simulink library "sm_boom_lift_crawler_lib_actuators"  (R2026a)
settings: Solver=ode23t
undefined symbols (not defined in the file): actuators, BasketR, cylinders, Extend, Jib, LevelM, LevelS, Lift, lines, OutFL, OutFR, OutRL, OutRR, Tilt, TrackL, TrackR, Turret, valves
libraries: SimscapeFluids_lib x92, fl_lib x67, sm_boom_lift_crawler_lib x24, nesl_utility x13, Custom_Valves x2
(part 5 of 5)

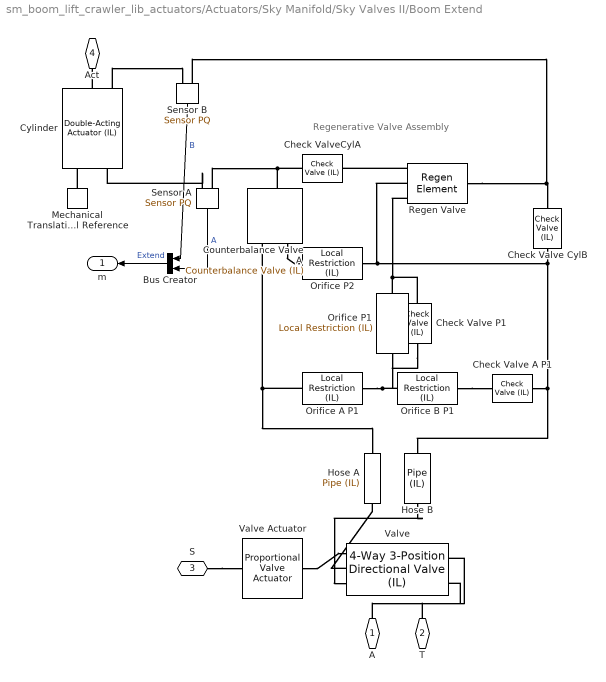
== system sm_boom_lift_crawler_lib_actuators/Actuators/Sky Manifold/Sky Valves II/Boom Extend ==
  note: Regenerative Valve Assembly
  Bus Creator : BusCreator  Inputs=2
  Check Valve P1 : SimscapeFluids_lib/Isothermal Liquid/Valves & Orifices/Directional Control Valves/Check Valve (IL)  opening_spec=fluids.isothermal_liquid.valves_orifices.enum.PressureOpeningSpec.Linear  pressure_control_spec=fluids.isothermal_liquid.valves_orifices.enum.pressure_control_spec.dp  p_crack_differential=valves.check.p.crack psi  p_crack_gauge=0.1 MPa  press_max_differential=valves.check.p.max psi  press_max_gauge=0.2 MPa  area_max=orifices.sky.rg.s in^2  area_leak=1e-12 m^2  p_diff_TLU=[0.01 : 0.01 : 0.1] MPa  valve_area_TLU=[1e-10, 1e-05, 2e-05, 3e-05, 4e-05, 5e-05, 6e-05, 7.5e-05, 8.5e-05, .0001] m^2  vol_flow_TLU=[.000358, .045, .11, .191, .284, .39, .505, .63, .764, .905] .* 1e-3 m^3/s  area=inf m^2  Cd=0.7  Re_c=150  smoothing_factor=0  pressure_recovery=false  opening_dynamics=1  tau=0.1 s
  Check Valve A P1 : SimscapeFluids_lib/Isothermal Liquid/Valves & Orifices/Directional Control Valves/Check Valve (IL)  opening_spec=fluids.isothermal_liquid.valves_orifices.enum.PressureOpeningSpec.Linear  pressure_control_spec=fluids.isothermal_liquid.valves_orifices.enum.pressure_control_spec.dp  p_crack_differential=valves.check.p.crack psi  p_crack_gauge=0.1 MPa  press_max_differential=valves.check.p.max psi  press_max_gauge=0.2 MPa  area_max=orifices.sky.r2.s in^2  area_leak=1e-12 m^2  p_diff_TLU=[0.01 : 0.01 : 0.1] MPa  valve_area_TLU=[1e-10, 1e-05, 2e-05, 3e-05, 4e-05, 5e-05, 6e-05, 7.5e-05, 8.5e-05, .0001] m^2  vol_flow_TLU=[.000358, .045, .11, .191, .284, .39, .505, .63, .764, .905] .* 1e-3 m^3/s  area=inf m^2  Cd=0.7  Re_c=150  smoothing_factor=0  pressure_recovery=false  opening_dynamics=1  tau=0.1 s
  Check Valve CylB : SimscapeFluids_lib/Isothermal Liquid/Valves & Orifices/Directional Control Valves/Check Valve (IL)  opening_spec=fluids.isothermal_liquid.valves_orifices.enum.PressureOpeningSpec.Linear  pressure_control_spec=fluids.isothermal_liquid.valves_orifices.enum.pressure_control_spec.dp  p_crack_differential=valves.check.p.crack psi  p_crack_gauge=0.1 MPa  press_max_differential=valves.check.p.max psi  press_max_gauge=0.2 MPa  area_max=lines.sky.c3.d.b in^2  area_leak=1e-12 m^2  p_diff_TLU=[0.01 : 0.01 : 0.1] MPa  valve_area_TLU=[1e-10, 1e-05, 2e-05, 3e-05, 4e-05, 5e-05, 6e-05, 7.5e-05, 8.5e-05, .0001] m^2  vol_flow_TLU=[.000358, .045, .11, .191, .284, .39, .505, .63, .764, .905] .* 1e-3 m^3/s  area=inf m^2  Cd=0.7  Re_c=150  smoothing_factor=0  pressure_recovery=false  opening_dynamics=0  tau=0.1 s
  Check ValveCylA : SimscapeFluids_lib/Isothermal Liquid/Valves & Orifices/Directional Control Valves/Check Valve (IL)  opening_spec=fluids.isothermal_liquid.valves_orifices.enum.PressureOpeningSpec.Linear  pressure_control_spec=fluids.isothermal_liquid.valves_orifices.enum.pressure_control_spec.dp  p_crack_differential=valves.check.p.crack psi  p_crack_gauge=0.1 MPa  press_max_differential=valves.check.p.max psi  press_max_gauge=0.2 MPa  area_max=lines.sky.c3.s.a in^2  area_leak=1e-12 m^2  p_diff_TLU=[0.01 : 0.01 : 0.1] MPa  valve_area_TLU=[1e-10, 1e-05, 2e-05, 3e-05, 4e-05, 5e-05, 6e-05, 7.5e-05, 8.5e-05, .0001] m^2  vol_flow_TLU=[.000358, .045, .11, .191, .284, .39, .505, .63, .764, .905] .* 1e-3 m^3/s  area=inf m^2  Cd=0.7  Re_c=150  smoothing_factor=0  pressure_recovery=false  opening_dynamics=1  tau=0.1 s
  Counterbalance Valve A : SimscapeFluids_lib/Isothermal Liquid/Valves & Orifices/Pressure Control Valves/Counterbalance Valve (IL)  opening_spec=1  p_set_diff=valves.counterbalance.c3.ps psi  p_max_diff=(valves.counterbalance.c3.k)*(valves.control.l.max) + (valves.counterbalance.c3.ps) psi  area_max=lines.sky.c3.s.a in^2  area_leak=1e-9 in^2  p_diff_TLU=39.3701*(valves.counterbalance.c3.k)*([-.002, 0, .005, .015]) + (valves.counterbalance.c3.ps) psi  valve_area_TLU=[1e-09, 4e-09, 1e-05, 1.02e-05] m^2  p_diff_TLU_ref=5 : 0.2 : 6 MPa  vol_flow_TLU_ref=[6.4e-09, .0013, .0027, .0041, .0055, .007] m^3/s  pilot_ratio=valves.counterbalance.c3.pr  back_ratio=valves.counterbalance.c3.pbr  Cd=0.7  Re_c=150  smoothing_factor=0  opening_dynamics=1  tau=valves.counterbalance.common.tau s  check_p_crack=valves.counterbalance.common.pc psi  check_p_max=valves.counterbalance.common.pm psi  check_area_max=lines.sky.c3.s.a in^2  check_p_diff_TLU=[0.01 : 0.01 : 0.1] MPa  check_area_TLU=[1e-10, 1e-05, 2e-05, 3e-05, 4e-05, 5e-05, 6e-05, 7.5e-05, 8.5e-05, .0001] m^2  check_vol_flow_TLU=[.000358, .045, .11, .191, .284, .39, .505, .63, .764, .905] .* 1e-3 m^3/s
  Cylinder : SimscapeFluids_lib/Isothermal Liquid/Actuators/Double-Acting Actuator (IL)  single_fluid=true  mech_orientation=1  piston_area_A=cylinders.sky.c3.s.a in^2  piston_area_B=cylinders.sky.c3.s.b in^2  stroke=cylinders.sky.c3.stroke in  dead_volume_A=cylinders.sky.c3.v.dead in^3  dead_volume_B=cylinders.sky.c3.v.dead in^3  pressure_spec=foundation.enum.pressure_spec.atmospheric  environment_pressure=0.101325 MPa  hardstop_model=1  stiff_coeff=cylinders.sky.c3.stops.kc N/m  damping_coeff=cylinders.sky.c3.stops.bc N/(m/s)  transition=1 mm  coeff_rest=0.7  v_tol=0.001 m/s  f_tol=0.001 N  cushion_A_spec=false  area_plunger_A=1e-4 m^2  length_plunger_A=1e-3 m  area_cushion_orifice_A=1e-6 m^2  area_leak_plunger_A=1e-7 m^2  p_crack_differential_A=0.01 MPa  press_max_differential_A=0.1 MPa  check_valve_area_max_A=1e-4 m^2  check_valve_area_leak_A=1e-10 m^2  smoothing_factor_A=0  cushion_B_spec=false  area_plunger_B=1e-4 m^2  length_plunger_B=1e-3 m  area_cushion_orifice_B=1e-6 m^2  area_leak_plunger_B=1e-7 m^2  p_crack_differential_B=0.01 MPa  press_max_differential_B=0.1 MPa  check_valve_area_max_B=1e-4 m^2  check_valve_area_leak_B=1e-10 m^2  smoothing_factor_B=0  friction_spec=false  breakaway_Coulomb_ratio=1.2  breakaway_velocity=0.1 m/s  preload_force=20 N  Coulomb_coeff=1e-6 N/Pa  viscous_coeff=100 N*s/m  leakage_spec=false  clearance=1e-4 m  piston_length=0.01 m  displacement_spec=foundation.enum.DisplacementSpec.Calculate  x0=0 in  dynamic_compressibility=true  p0_A=lines.sky.c3.p0.a + 14.6959 psi  p0_B=lines.sky.c3.p0.b + 14.6959 psi  p_nominal_A=0.101325 MPa  p_nominal_B=0.101325 MPa
      settings: LogSimulationData=on
  Hose A : SimscapeFluids_lib/Isothermal Liquid/Pipes & Fittings/Pipe (IL)  dynamic_compressibility=true  inertia=false  num_segments=1  pipe_length=lines.sky.c3.l ft  cross_section_geometry=fluids.isothermal_liquid.pipes_fittings.enum.cross_section_geometry.circular  pipe_diameter=lines.sky.c3.d.a in  pipe_inner_diameter=0.05 m  pipe_outer_diameter=0.1 m  pipe_width=0.1 m  pipe_height=0.1 m  pipe_major_axis=0.1 m  pipe_minor_axis=0.05 m  pipe_side=0.1 m  pipe_angle=30 deg  pipe_area=1e-4 m^2  Dh=1.12e-2 m  elevation_spec=foundation.enum.constant_variable.constant  elevation_gain=0 m  gravity_spec=foundation.enum.constant_variable.constant  g=9.81 m/s^2  pressure_loss_spec=fluids.isothermal_liquid.pipes_fittings.enum.pressure_loss_spec.haaland  mdot_nominal=[.1, 1] kg/s  p_diff_nominal=[.001, .01] MPa  mdot_threshold=1e-6 kg/s  local_pressure_loss_spec=fluids.isothermal_liquid.pipes_fittings.enum.local_loss_spec.aggregate_length  length_add=lines.sky.c3.lr ft  loss_coefficient=0.1  roughness_spec=fluids.isothermal_liquid.pipes_fittings.enum.roughness_spec.custom  roughness=15e-6 m  Re_friction_TLU=[400, 1000, 1500, 3000, 4000, 6000, 10000, 20000, 40000, 60000, 100000, 100000000]  friction_factor_TLU=[.264, .112, .071, .0417, .0387, .0268, .025, .0232, .0226, .022, .0214, .0214]  Re_lam=2000  Re_tur=4000  shape_factor=64  pipe_wall_spec=fluids.isothermal_liquid.pipes_fittings.enum.wall_spec.rigid  vol_expansion_spec=fluids.isothermal_liquid.pipes_fittings.enum.vol_expansion_spec.area  area_pressure_gain=1e-6 m^2/MPa  static_pressure_TLU=[.1, 1] MPa  area_pressure_gain_TLU=[1e-05, 1.1e-05] m^2  material_behavior_spec=fluids.isothermal_liquid.pipes_fittings.enum.PipeMaterialBehavior.Linear  diameter_pressure_gain=2e-12 m/Pa  wall_thickness=0.05 m  elastic_modulus=69 GPa  stress_TLU=[276, 310] MPa  strain_TLU=[.004, .02]  stress_assert_action=simscape.enum.assert.action.none  stress_max=400 MPa  poisson_ratio=0.33  wall_time_constant=0.01 s  p0=lines.sky.c3.p0.a + 14.6959 psi  mdot0=0 kg/s
  Hose B : SimscapeFluids_lib/Isothermal Liquid/Pipes & Fittings/Pipe (IL)  dynamic_compressibility=true  inertia=false  num_segments=1  pipe_length=lines.sky.c3.l ft  cross_section_geometry=fluids.isothermal_liquid.pipes_fittings.enum.cross_section_geometry.circular  pipe_diameter=lines.sky.c3.d.b in  pipe_inner_diameter=0.05 m  pipe_outer_diameter=0.1 m  pipe_width=0.1 m  pipe_height=0.1 m  pipe_major_axis=0.1 m  pipe_minor_axis=0.05 m  pipe_side=0.1 m  pipe_angle=30 deg  pipe_area=1e-4 m^2  Dh=1.12e-2 m  elevation_spec=foundation.enum.constant_variable.constant  elevation_gain=0 m  gravity_spec=foundation.enum.constant_variable.constant  g=9.81 m/s^2  pressure_loss_spec=fluids.isothermal_liquid.pipes_fittings.enum.pressure_loss_spec.haaland  mdot_nominal=[.1, 1] kg/s  p_diff_nominal=[.001, .01] MPa  mdot_threshold=1e-6 kg/s  local_pressure_loss_spec=fluids.isothermal_liquid.pipes_fittings.enum.local_loss_spec.aggregate_length  length_add=lines.sky.c3.lr ft  loss_coefficient=0.1  roughness_spec=fluids.isothermal_liquid.pipes_fittings.enum.roughness_spec.custom  roughness=15e-6 m  Re_friction_TLU=[400, 1000, 1500, 3000, 4000, 6000, 10000, 20000, 40000, 60000, 100000, 100000000]  friction_factor_TLU=[.264, .112, .071, .0417, .0387, .0268, .025, .0232, .0226, .022, .0214, .0214]  Re_lam=2000  Re_tur=4000  shape_factor=64  pipe_wall_spec=fluids.isothermal_liquid.pipes_fittings.enum.wall_spec.rigid  vol_expansion_spec=fluids.isothermal_liquid.pipes_fittings.enum.vol_expansion_spec.area  area_pressure_gain=1e-6 m^2/MPa  static_pressure_TLU=[.1, 1] MPa  area_pressure_gain_TLU=[1e-05, 1.1e-05] m^2  material_behavior_spec=fluids.isothermal_liquid.pipes_fittings.enum.PipeMaterialBehavior.Linear  diameter_pressure_gain=2e-12 m/Pa  wall_thickness=0.05 m  elastic_modulus=69 GPa  stress_TLU=[276, 310] MPa  strain_TLU=[.004, .02]  stress_assert_action=simscape.enum.assert.action.none  stress_max=400 MPa  poisson_ratio=0.33  wall_time_constant=0.01 s  p0=lines.sky.c3.p0.b + 14.6959 psi  mdot0=0 kg/s
  Mechanical Translational Reference : fl_lib/Mechanical/Translational Elements/Mechanical Translational Reference
  Orifice A P1 : fl_lib/Isothermal Liquid/Elements/Local Restriction (IL)  restriction_type=1  restriction_area=orifices.sky.rg.s in^2  min_area=1e-10 m^2  max_area=0.005 m^2  area=inf in^2  Cd=0.7  Re_c=150  pressure_recovery=simscape.enum.onoff.off
  Orifice B P1 : fl_lib/Isothermal Liquid/Elements/Local Restriction (IL)  restriction_type=1  restriction_area=orifices.sky.rg.s in^2  min_area=1e-10 m^2  max_area=0.005 m^2  area=inf in^2  Cd=0.7  Re_c=150  pressure_recovery=simscape.enum.onoff.off
  Orifice P1 : fl_lib/Isothermal Liquid/Elements/Local Restriction (IL)  restriction_type=1  restriction_area=orifices.sky.rg.s in^2  min_area=1e-10 m^2  max_area=0.005 m^2  area=inf in^2  Cd=0.7  Re_c=150  pressure_recovery=simscape.enum.onoff.off
  Orifice P2 : fl_lib/Isothermal Liquid/Elements/Local Restriction (IL)  restriction_type=1  restriction_area=orifices.sky.rg.s in^2  min_area=1e-10 m^2  max_area=0.005 m^2  area=inf in^2  Cd=0.7  Re_c=150  pressure_recovery=simscape.enum.onoff.off
  Regen Valve : Custom_Valves/Regen Element  sMax=valves.control.l.max  T=0.1  pCrack=1450  pMax=1550  AMax=lines.sky.c3.s.a  kA=1  kP1=3  kP2=1
  Sensor A : sm_boom_lift_crawler_lib/Sensor PQ  SystemSampleTime=-1  VariantActivationTime=update diagram  EmptyChoice=off  PassThrough=off  PassThroughVariantControl=(default)  EmptyChoiceVariantControl=(default)  AllowFlexibleInterface=on  Latency=0  AutoFrameSizeCalculation=off
  Sensor B : sm_boom_lift_crawler_lib/Sensor PQ  SystemSampleTime=-1  VariantActivationTime=update diagram  EmptyChoice=off  PassThrough=off  PassThroughVariantControl=(default)  EmptyChoiceVariantControl=(default)  AllowFlexibleInterface=on  Latency=0  AutoFrameSizeCalculation=off
  Valve : SimscapeFluids_lib/Isothermal Liquid/Valves & Orifices/Directional Control Valves/4-Way 3-Position Directional Valve (IL)  open_orifices_pos=fluids.isothermal_liquid.valves_orifices.directional_control_valves.enum.directional_valve_open_orifices_pos_neg.PA_BT  open_orifices_neu=fluids.isothermal_liquid.valves_orifices.directional_control_valves.enum.directional_valve_open_orifices_neutral.all_closed  open_orifices_neg=fluids.isothermal_liquid.valves_orifices.directional_control_valves.enum.directional_valve_open_orifices_pos_neg.PB_AT  neutral_assert_action=0  area_spec=fluids.isothermal_liquid.valves_orifices.directional_control_valves.enum.directional_valve_area_spec.different  valve_spec=1  del_S_max=(valves.control.l.max) - (valves.control.l.max)/(lines.sky.r1.s)*(1e-9) in  area_max=lines.sky.r1.s in^2  del_S_TLU=[0, .00125, .0025, .00375, .005] m  valve_area_TLU=[1e-09, 2.0352e-07, 4.0736e-05, .00011438, .00034356] m^2  del_S_vol_flow_TLU=[0, .00125, .0025, .00375, .005] m  p_diff_TLU=[-10000000, -5000000, -2000000, 2000000, 5000000, 10000000] Pa  vol_flow_TLU=[-1e-07, -7.0711e-08, -4.4721e-08, 4.4721e-08, 7.0711e-08, 1e-07; -2.0352e-05, -1.4391e-05, -9.1017e-06, 9.1017e-06, 1.4391e-05, 2.0352e-05; -.0040736, -.0028805, -.0018218, .0018218, .0028805, .0040736; -.011438, -.0080879, -.0051152, .0051152, .0080879, .011438; -.034356, -.024293, -.015364, .015364, .024293, .034356] m^3/s  p_diff_TLU_const=[-.1, .3, .5, .7] MPa  vol_flow_TLU_const=[-.0009, .0016, .002, .0024] m^3/s  area_const=1e-4 m^2  area_leak=1e-9 in^2  area=inf m^2  Cd=0.7  Re_c=150  smoothing_factor=0.01  pressure_recovery=false  S_max_PA=-(0) + 0.0254*(valves.control.l.max) m  del_S_max_PA=(valves.control.l.max) - (valves.control.l.max)/(lines.sky.c3.s.a)*(1e-9) in  area_max_PA=lines.sky.c3.s.a in^2  del_S_TLU_PA=[0, .00125, .0025, .00375, .005] m  valve_area_TLU_PA=[1e-09, 2.0352e-07, 4.0736e-05, .00011438, .00034356] m^2  del_S_vol_flow_TLU_PA=[0, .00125, .0025, .00375, .005] m  p_diff_TLU_PA=[-10000000, -5000000, -2000000, 2000000, 5000000, 10000000] Pa  vol_flow_TLU_PA=[-1e-07, -7.0711e-08, -4.4721e-08, 4.4721e-08, 7.0711e-08, 1e-07; -2.0352e-05, -1.4391e-05, -9.1017e-06, 9.1017e-06, 1.4391e-05, 2.0352e-05; -.0040736, -.0028805, -.0018218, .0018218, .0028805, .0040736; -.011438, -.0080879, -.0051152, .0051152, .0080879, .011438; -.034356, -.024293, -.015364, .015364, .024293, .034356] m^3/s  area_const_PA=1e-4 m^2  p_diff_TLU_const_PA=[-.1, .3, .5, .7] MPa  vol_flow_TLU_const_PA=[-.0009, .0016, .002, .0024] m^3/s  S_max_PB=(0) - 0.0254*(valves.control.l.max) m  del_S_max_PB=(valves.control.l.max) - (valves.control.l.max)/(lines.sky.c3.s.b)*(1e-9) in  area_max_PB=lines.sky.c3.s.b in^2  del_S_TLU_PB=[0, .00125, .0025, .00375, .005] m  valve_area_TLU_PB=[1e-09, 2.0352e-07, 4.0736e-05, .00011438, .00034356] m^2  del_S_vol_flow_TLU_PB=[0, .00125, .0025, .00375, .005] m  p_diff_TLU_PB=[-10000000, -5000000, -2000000, 2000000, 5000000, 10000000] Pa  vol_flow_TLU_PB=[-1e-07, -7.0711e-08, -4.4721e-08, 4.4721e-08, 7.0711e-08, 1e-07; -2.0352e-05, -1.4391e-05, -9.1017e-06, 9.1017e-06, 1.4391e-05, 2.0352e-05; -.0040736, -.0028805, -.0018218, .0018218, .0028805, .0040736; -.011438, -.0080879, -.0051152, .0051152, .0080879, .011438; -.034356, -.024293, -.015364, .015364, .024293, .034356] m^3/s  area_const_PB=1e-4 m^2  p_diff_TLU_const_PB=[-.1, .3, .5, .7] MPa  vol_flow_TLU_const_PB=[-.0009, .0016, .002, .0024] m^3/s  S_max_AB=7.5e-3 m  del_S_max_AB=0.005 m  area_max_AB=1e-4 m^2  del_S_TLU_AB=[0, .00125, .0025, .00375, .005] m  valve_area_TLU_AB=[1e-10, 1e-05, 4e-05, 6e-05, .0001] m^2  del_S_vol_flow_TLU_AB=[0, .00125, .0025, .00375, .005] m  p_diff_TLU_AB=[-.1, .3, .5, .7] MPa  vol_flow_TLU_AB=[-1e-08, 2.2e-08, 2.8e-08, 3.4e-08; -9e-06, .00015, .0002, .00024; -.00036, .00063, .00081, .00096; -.00054, .00094, .0012, .0014; -.00091, .0016, .002, .0024] m^3/s  area_const_AB=1e-4 m^2  p_diff_TLU_const_AB=[-.1, .3, .5, .7] MPa  vol_flow_TLU_const_AB=[-.0009, .0016, .002, .0024] m^3/s  S_max_AT=(0) - 0.0254*(valves.control.l.max) m  del_S_max_AT=(valves.control.l.max) - (valves.control.l.max)/(lines.sky.main.s.t)*(1e-9) in  area_max_AT=lines.sky.main.s.t in^2  del_S_TLU_AT=[0, .00125, .0025, .00375, .005] m  valve_area_TLU_AT=[1e-09, 2.0352e-07, 4.0736e-05, .00011438, .00034356] m^2  del_S_vol_flow_TLU_AT=[0, .00125, .0025, .00375, .005] m  p_diff_TLU_AT=[-10000000, -5000000, -2000000, 2000000, 5000000, 10000000] Pa  vol_flow_TLU_AT=[-1e-07, -7.0711e-08, -4.4721e-08, 4.4721e-08, 7.0711e-08, 1e-07; -2.0352e-05, -1.4391e-05, -9.1017e-06, 9.1017e-06, 1.4391e-05, 2.0352e-05; -.0040736, -.0028805, -.0018218, .0018218, .0028805, .0040736; -.011438, -.0080879, -.0051152, .0051152, .0080879, .011438; -.034356, -.024293, -.015364, .015364, .024293, .034356] m^3/s  area_const_AT=1e-4 m^2  p_diff_TLU_const_AT=[-.1, .3, .5, .7] MPa  vol_flow_TLU_const_AT=[-.0009, .0016, .002, .0024] m^3/s  S_max_BT=-(0) + 0.0254*(valves.control.l.max) m  del_S_max_BT=(valves.control.l.max) - (valves.control.l.max)/(lines.sky.main.s.t)*(1e-9) in  area_max_BT=lines.sky.main.s.t in^2  del_S_TLU_BT=[0, .00125, .0025, .00375, .005] m  valve_area_TLU_BT=[1e-09, 2.0352e-07, 4.0736e-05, .00011438, .00034356] m^2  del_S_vol_flow_TLU_BT=[0, .00125, .0025, .00375, .005] m  p_diff_TLU_BT=[-10000000, -5000000, -2000000, 2000000, 5000000, 10000000] Pa  vol_flow_TLU_BT=[-1e-07, -7.0711e-08, -4.4721e-08, 4.4721e-08, 7.0711e-08, 1e-07; -2.0352e-05, -1.4391e-05, -9.1017e-06, 9.1017e-06, 1.4391e-05, 2.0352e-05; -.0040736, -.0028805, -.0018218, .0018218, .0028805, .0040736; -.011438, -.0080879, -.0051152, .0051152, .0080879, .011438; -.034356, -.024293, -.015364, .015364, .024293, .034356] m^3/s  area_const_BT=1e-4 m^2  p_diff_TLU_const_BT=[-.1, .3, .5, .7] MPa  vol_flow_TLU_const_BT=[-.0009, .0016, .002, .0024] m^3/s  S_max_PT=0 m  del_S_max_PT=0.005 m  area_max_PT=1e-4 m^2  del_S_TLU_PT=[0, .00125, .0025, .00375, .005] m  valve_area_TLU_PT=[1e-10, 1e-05, 4e-05, 6e-05, .0001] m^2  del_S_vol_flow_TLU_PT=[0, .00125, .0025, .00375, .005] m  p_diff_TLU_PT=[-.1, .3, .5, .7] MPa  vol_flow_TLU_PT=[-1e-08, 2.2e-08, 2.8e-08, 3.4e-08; -9e-06, .00015, .0002, .00024; -.00036, .00063, .00081, .00096; -.00054, .00094, .0012, .0014; -.00091, .0016, .002, .0024] m^3/s
  Valve Actuator : SimscapeFluids_lib/Valve Actuators/Proportional Valve Actuator  gain=1 in  time_constant=valves.control.tau.b s  valve_stroke=valves.control.l.max in
  A : PMIOPort  Side=Right
  T : PMIOPort  Port=2  Side=Right
  S : PMIOPort  Port=3  Side=Left
  Act : PMIOPort  Port=4  Side=Left
  m : Outport
  wires:
  Bus Creator/1 -> m/1  "Extend"
  Sensor A/1 -> Bus Creator/2  "A"
  Sensor B/1 -> Bus Creator/1  "B"
  connections:
  T/RConn1 -- Valve/RConn2
  A/RConn1 -- Valve/RConn1
  Valve Actuator/RConn1 -- Valve/LConn1
  Regen Valve/RConn1 -- Check ValveCylA/LConn1
  Orifice A P1/RConn1 -- Check Valve P1/RConn1 -- Orifice P1/LConn1 -- Orifice B P1/RConn1
  Orifice B P1/LConn1 -- Check Valve A P1/LConn1
  Regen Valve/LConn1 -- Sensor B/LConn2 -- Check Valve CylB/RConn1
  Orifice P2/RConn1 -- Check Valve CylB/LConn1 -- Check Valve A P1/RConn1 -- Hose B/RConn1 -- Regen Valve/RConn2
  S/RConn1 -- Valve Actuator/LConn1
  Counterbalance Valve A/LConn1 -- Check ValveCylA/RConn1 -- Sensor A/LConn2
  Cylinder/RConn2 -- Act/RConn1
  Cylinder/RConn3 -- Sensor B/LConn1
  Mechanical Translational Reference/LConn1 -- Cylinder/LConn1
  Sensor A/LConn1 -- Cylinder/LConn2
  Orifice A P1/LConn1 -- Counterbalance Valve A/RConn2 -- Hose A/RConn1
  Orifice P1/RConn1 -- Regen Valve/RConn3 -- Check Valve P1/LConn1
  Counterbalance Valve A/RConn1 -- Orifice P2/LConn1
  Hose B/LConn1 -- Valve/LConn3
  Valve/LConn2 -- Hose A/LConn1

== system sm_boom_lift_crawler_lib_actuators/Actuators/Sky Manifold/Sky Valves II/Jib Lift ==
  Bus Creator : BusCreator  Inputs=2
  CVHC CbValveBB : fl_lib/Isothermal Liquid/Elements/Constant Volume Chamber (IL)  Commented=on  volume=1e-4 m^3  p_I_specify=off  p_I_priority=High  p_I=0.101325 MPa  p_I_nominal_specify=off  p_I_nominal_value=1  p_I_nominal_unit=MPa
  CVHC CbValveBP : fl_lib/Isothermal Liquid/Elements/Constant Volume Chamber (IL)  Commented=on  volume=1e-4 m^3  p_I_specify=off  p_I_priority=High  p_I=0.101325 MPa  p_I_nominal_specify=off  p_I_nominal_value=1  p_I_nominal_unit=MPa
  Counterbalance Valve A : SimscapeFluids_lib/Isothermal Liquid/Valves & Orifices/Pressure Control Valves/Counterbalance Valve (IL)  opening_spec=1  p_set_diff=valves.counterbalance.c4.ps.ii psi  p_max_diff=(valves.counterbalance.c4.k)*(valves.control.l.max) + (valves.counterbalance.c4.ps.ii) psi  area_max=lines.sky.c4.s in^2  area_leak=1e-9 in^2  p_diff_TLU=39.3701*(valves.counterbalance.c4.k)*([-.002, 0, .005, .015]) + (valves.counterbalance.c4.ps.ii) psi  valve_area_TLU=[1e-09, 4e-09, 1e-05, 1.02e-05] m^2  p_diff_TLU_ref=5 : 0.2 : 6 MPa  vol_flow_TLU_ref=[6.4e-09, .0013, .0027, .0041, .0055, .007] m^3/s  pilot_ratio=valves.counterbalance.c4.pr.ii  back_ratio=valves.counterbalance.c4.pbr  Cd=0.7  Re_c=150  smoothing_factor=0.001  opening_dynamics=1  tau=valves.counterbalance.common.tau s  check_p_crack=valves.counterbalance.common.pc psi  check_p_max=valves.counterbalance.common.pm psi  check_area_max=lines.sky.c4.s in^2  check_p_diff_TLU=[0.01 : 0.01 : 0.1] MPa  check_area_TLU=[1e-10, 1e-05, 2e-05, 3e-05, 4e-05, 5e-05, 6e-05, 7.5e-05, 8.5e-05, .0001] m^2  check_vol_flow_TLU=[.000358, .045, .11, .191, .284, .39, .505, .63, .764, .905] .* 1e-3 m^3/s
  Counterbalance Valve B : SimscapeFluids_lib/Isothermal Liquid/Valves & Orifices/Pressure Control Valves/Counterbalance Valve (IL)  opening_spec=1  p_set_diff=valves.counterbalance.c4.ps.i psi  p_max_diff=(valves.counterbalance.c4.k)*(valves.control.l.max) + (valves.counterbalance.c4.ps.i) psi  area_max=lines.sky.c4.s in^2  area_leak=1e-9 in^2  p_diff_TLU=39.3701*(valves.counterbalance.c4.k)*([-.002, 0, .005, .015]) + (valves.counterbalance.c4.ps.i) psi  valve_area_TLU=[1e-09, 4e-09, 1e-05, 1.02e-05] m^2  p_diff_TLU_ref=5 : 0.2 : 6 MPa  vol_flow_TLU_ref=[6.4e-09, .0013, .0027, .0041, .0055, .007] m^3/s  pilot_ratio=valves.counterbalance.c4.pr.i  back_ratio=valves.counterbalance.c4.pbr  Cd=0.7  Re_c=150  smoothing_factor=0.001  opening_dynamics=1  tau=valves.counterbalance.common.tau s  check_p_crack=valves.counterbalance.common.pc psi  check_p_max=valves.counterbalance.common.pm psi  check_area_max=lines.sky.c4.s in^2  check_p_diff_TLU=[0.01 : 0.01 : 0.1] MPa  check_area_TLU=[1e-10, 1e-05, 2e-05, 3e-05, 4e-05, 5e-05, 6e-05, 7.5e-05, 8.5e-05, .0001] m^2  check_vol_flow_TLU=[.000358, .045, .11, .191, .284, .39, .505, .63, .764, .905] .* 1e-3 m^3/s
  Cylinder : SimscapeFluids_lib/Isothermal Liquid/Actuators/Double-Acting Actuator (IL)  single_fluid=true  mech_orientation=1  piston_area_A=cylinders.sky.c4.s.a in^2  piston_area_B=cylinders.sky.c4.s.b in^2  stroke=cylinders.sky.c4.stroke in  dead_volume_A=cylinders.sky.c4.v.dead in^3  dead_volume_B=cylinders.sky.c4.v.dead in^3  pressure_spec=foundation.enum.pressure_spec.atmospheric  environment_pressure=0.101325 MPa  hardstop_model=1  stiff_coeff=cylinders.sky.c4.stops.kc N/m  damping_coeff=cylinders.sky.c4.stops.bc N/(m/s)  transition=1 mm  coeff_rest=0.7  v_tol=0.001 m/s  f_tol=0.001 N  cushion_A_spec=false  area_plunger_A=1e-4 m^2  length_plunger_A=1e-3 m  area_cushion_orifice_A=1e-6 m^2  area_leak_plunger_A=1e-7 m^2  p_crack_differential_A=0.01 MPa  press_max_differential_A=0.1 MPa  check_valve_area_max_A=1e-4 m^2  check_valve_area_leak_A=1e-10 m^2  smoothing_factor_A=0  cushion_B_spec=false  area_plunger_B=1e-4 m^2  length_plunger_B=1e-3 m  area_cushion_orifice_B=1e-6 m^2  area_leak_plunger_B=1e-7 m^2  p_crack_differential_B=0.01 MPa  press_max_differential_B=0.1 MPa  check_valve_area_max_B=1e-4 m^2  check_valve_area_leak_B=1e-10 m^2  smoothing_factor_B=0  friction_spec=false  breakaway_Coulomb_ratio=1.2  breakaway_velocity=0.1 m/s  preload_force=20 N  Coulomb_coeff=1e-6 N/Pa  viscous_coeff=100 N*s/m  leakage_spec=false  clearance=1e-4 m  piston_length=0.01 m  displacement_spec=foundation.enum.DisplacementSpec.Calculate  x0=0 in  dynamic_compressibility=true  p0_A=lines.sky.c4.p0.a + 14.6959 psi  p0_B=lines.sky.c4.p0.b + 14.6959 psi  p_nominal_A=0.101325 MPa  p_nominal_B=0.101325 MPa
      settings: LogSimulationData=on
  Hose A : SimscapeFluids_lib/Isothermal Liquid/Pipes & Fittings/Pipe (IL)  dynamic_compressibility=true  inertia=false  num_segments=1  pipe_length=lines.sky.c4.l ft  cross_section_geometry=fluids.isothermal_liquid.pipes_fittings.enum.cross_section_geometry.circular  pipe_diameter=lines.sky.c4.d in  pipe_inner_diameter=0.05 m  pipe_outer_diameter=0.1 m  pipe_width=0.1 m  pipe_height=0.1 m  pipe_major_axis=0.1 m  pipe_minor_axis=0.05 m  pipe_side=0.1 m  pipe_angle=30 deg  pipe_area=1e-4 m^2  Dh=1.12e-2 m  elevation_spec=foundation.enum.constant_variable.constant  elevation_gain=0 m  gravity_spec=foundation.enum.constant_variable.constant  g=9.81 m/s^2  pressure_loss_spec=fluids.isothermal_liquid.pipes_fittings.enum.pressure_loss_spec.haaland  mdot_nominal=[.1, 1] kg/s  p_diff_nominal=[.001, .01] MPa  mdot_threshold=1e-6 kg/s  local_pressure_loss_spec=fluids.isothermal_liquid.pipes_fittings.enum.local_loss_spec.aggregate_length  length_add=lines.sky.c4.lr ft  loss_coefficient=0.1  roughness_spec=fluids.isothermal_liquid.pipes_fittings.enum.roughness_spec.custom  roughness=15e-6 m  Re_friction_TLU=[400, 1000, 1500, 3000, 4000, 6000, 10000, 20000, 40000, 60000, 100000, 100000000]  friction_factor_TLU=[.264, .112, .071, .0417, .0387, .0268, .025, .0232, .0226, .022, .0214, .0214]  Re_lam=2000  Re_tur=4000  shape_factor=64  pipe_wall_spec=fluids.isothermal_liquid.pipes_fittings.enum.wall_spec.rigid  vol_expansion_spec=fluids.isothermal_liquid.pipes_fittings.enum.vol_expansion_spec.area  area_pressure_gain=1e-6 m^2/MPa  static_pressure_TLU=[.1, 1] MPa  area_pressure_gain_TLU=[1e-05, 1.1e-05] m^2  material_behavior_spec=fluids.isothermal_liquid.pipes_fittings.enum.PipeMaterialBehavior.Linear  diameter_pressure_gain=2e-12 m/Pa  wall_thickness=0.05 m  elastic_modulus=69 GPa  stress_TLU=[276, 310] MPa  strain_TLU=[.004, .02]  stress_assert_action=simscape.enum.assert.action.none  stress_max=400 MPa  poisson_ratio=0.33  wall_time_constant=0.01 s  p0=lines.sky.c4.p0.a + 14.6959 psi  mdot0=0 kg/s
  Hose B : SimscapeFluids_lib/Isothermal Liquid/Pipes & Fittings/Pipe (IL)  dynamic_compressibility=true  inertia=false  num_segments=1  pipe_length=lines.sky.c4.l ft  cross_section_geometry=fluids.isothermal_liquid.pipes_fittings.enum.cross_section_geometry.circular  pipe_diameter=lines.sky.c4.d in  pipe_inner_diameter=0.05 m  pipe_outer_diameter=0.1 m  pipe_width=0.1 m  pipe_height=0.1 m  pipe_major_axis=0.1 m  pipe_minor_axis=0.05 m  pipe_side=0.1 m  pipe_angle=30 deg  pipe_area=1e-4 m^2  Dh=1.12e-2 m  elevation_spec=foundation.enum.constant_variable.constant  elevation_gain=0 m  gravity_spec=foundation.enum.constant_variable.constant  g=9.81 m/s^2  pressure_loss_spec=fluids.isothermal_liquid.pipes_fittings.enum.pressure_loss_spec.haaland  mdot_nominal=[.1, 1] kg/s  p_diff_nominal=[.001, .01] MPa  mdot_threshold=1e-6 kg/s  local_pressure_loss_spec=fluids.isothermal_liquid.pipes_fittings.enum.local_loss_spec.aggregate_length  length_add=lines.sky.c4.lr ft  loss_coefficient=0.1  roughness_spec=fluids.isothermal_liquid.pipes_fittings.enum.roughness_spec.custom  roughness=15e-6 m  Re_friction_TLU=[400, 1000, 1500, 3000, 4000, 6000, 10000, 20000, 40000, 60000, 100000, 100000000]  friction_factor_TLU=[.264, .112, .071, .0417, .0387, .0268, .025, .0232, .0226, .022, .0214, .0214]  Re_lam=2000  Re_tur=4000  shape_factor=64  pipe_wall_spec=fluids.isothermal_liquid.pipes_fittings.enum.wall_spec.rigid  vol_expansion_spec=fluids.isothermal_liquid.pipes_fittings.enum.vol_expansion_spec.area  area_pressure_gain=1e-6 m^2/MPa  static_pressure_TLU=[.1, 1] MPa  area_pressure_gain_TLU=[1e-05, 1.1e-05] m^2  material_behavior_spec=fluids.isothermal_liquid.pipes_fittings.enum.PipeMaterialBehavior.Linear  diameter_pressure_gain=2e-12 m/Pa  wall_thickness=0.05 m  elastic_modulus=69 GPa  stress_TLU=[276, 310] MPa  strain_TLU=[.004, .02]  stress_assert_action=simscape.enum.assert.action.none  stress_max=400 MPa  poisson_ratio=0.33  wall_time_constant=0.01 s  p0=lines.sky.c4.p0.b + 14.6959 psi  mdot0=0 kg/s
  Mechanical Translational Reference : fl_lib/Mechanical/Translational Elements/Mechanical Translational Reference
  Sensor A : sm_boom_lift_crawler_lib/Sensor PQ  SystemSampleTime=-1  VariantActivationTime=update diagram  EmptyChoice=off  PassThrough=off  PassThroughVariantControl=(default)  EmptyChoiceVariantControl=(default)  AllowFlexibleInterface=on  Latency=0  AutoFrameSizeCalculation=off
  Sensor B : sm_boom_lift_crawler_lib/Sensor PQ  SystemSampleTime=-1  VariantActivationTime=update diagram  EmptyChoice=off  PassThrough=off  PassThroughVariantControl=(default)  EmptyChoiceVariantControl=(default)  AllowFlexibleInterface=on  Latency=0  AutoFrameSizeCalculation=off
  Valve : SimscapeFluids_lib/Isothermal Liquid/Valves & Orifices/Directional Control Valves/4-Way 3-Position Directional Valve (IL)  open_orifices_pos=fluids.isothermal_liquid.valves_orifices.directional_control_valves.enum.directional_valve_open_orifices_pos_neg.PA_BT  open_orifices_neu=fluids.isothermal_liquid.valves_orifices.directional_control_valves.enum.directional_valve_open_orifices_neutral.all_closed  open_orifices_neg=fluids.isothermal_liquid.valves_orifices.directional_control_valves.enum.directional_valve_open_orifices_pos_neg.PB_AT  neutral_assert_action=0  area_spec=fluids.isothermal_liquid.valves_orifices.directional_control_valves.enum.directional_valve_area_spec.different  valve_spec=1  del_S_max=(valves.control.l.max) - (valves.control.l.max)/(lines.sky.r1.s)*(1e-9) in  area_max=lines.sky.r1.s in^2  del_S_TLU=[0, .00125, .0025, .00375, .005] m  valve_area_TLU=[1e-09, 2.0352e-07, 4.0736e-05, .00011438, .00034356] m^2  del_S_vol_flow_TLU=[0, .00125, .0025, .00375, .005] m  p_diff_TLU=[-10000000, -5000000, -2000000, 2000000, 5000000, 10000000] Pa  vol_flow_TLU=[-1e-07, -7.0711e-08, -4.4721e-08, 4.4721e-08, 7.0711e-08, 1e-07; -2.0352e-05, -1.4391e-05, -9.1017e-06, 9.1017e-06, 1.4391e-05, 2.0352e-05; -.0040736, -.0028805, -.0018218, .0018218, .0028805, .0040736; -.011438, -.0080879, -.0051152, .0051152, .0080879, .011438; -.034356, -.024293, -.015364, .015364, .024293, .034356] m^3/s  p_diff_TLU_const=[-.1, .3, .5, .7] MPa  vol_flow_TLU_const=[-.0009, .0016, .002, .0024] m^3/s  area_const=1e-4 m^2  area_leak=1e-9 in^2  area=inf m^2  Cd=0.7  Re_c=150  smoothing_factor=0  pressure_recovery=false  S_max_PA=-(0) + 0.0254*(valves.control.l.max) m  del_S_max_PA=(valves.control.l.max) - (valves.control.l.max)/(lines.sky.c4.s)*(1e-9) in  area_max_PA=lines.sky.c4.s in^2  del_S_TLU_PA=[0, .00125, .0025, .00375, .005] m  valve_area_TLU_PA=[1e-09, 2.0352e-07, 4.0736e-05, .00011438, .00034356] m^2  del_S_vol_flow_TLU_PA=[0, .00125, .0025, .00375, .005] m  p_diff_TLU_PA=[-10000000, -5000000, -2000000, 2000000, 5000000, 10000000] Pa  vol_flow_TLU_PA=[-1e-07, -7.0711e-08, -4.4721e-08, 4.4721e-08, 7.0711e-08, 1e-07; -2.0352e-05, -1.4391e-05, -9.1017e-06, 9.1017e-06, 1.4391e-05, 2.0352e-05; -.0040736, -.0028805, -.0018218, .0018218, .0028805, .0040736; -.011438, -.0080879, -.0051152, .0051152, .0080879, .011438; -.034356, -.024293, -.015364, .015364, .024293, .034356] m^3/s  area_const_PA=1e-4 m^2  p_diff_TLU_const_PA=[-.1, .3, .5, .7] MPa  vol_flow_TLU_const_PA=[-.0009, .0016, .002, .0024] m^3/s  S_max_PB=(0) - 0.0254*(valves.control.l.max) m  del_S_max_PB=(valves.control.l.max) - (valves.control.l.max)/(lines.sky.c4.s)*(1e-9) in  area_max_PB=lines.sky.c4.s in^2  del_S_TLU_PB=[0, .00125, .0025, .00375, .005] m  valve_area_TLU_PB=[1e-09, 2.0352e-07, 4.0736e-05, .00011438, .00034356] m^2  del_S_vol_flow_TLU_PB=[0, .00125, .0025, .00375, .005] m  p_diff_TLU_PB=[-10000000, -5000000, -2000000, 2000000, 5000000, 10000000] Pa  vol_flow_TLU_PB=[-1e-07, -7.0711e-08, -4.4721e-08, 4.4721e-08, 7.0711e-08, 1e-07; -2.0352e-05, -1.4391e-05, -9.1017e-06, 9.1017e-06, 1.4391e-05, 2.0352e-05; -.0040736, -.0028805, -.0018218, .0018218, .0028805, .0040736; -.011438, -.0080879, -.0051152, .0051152, .0080879, .011438; -.034356, -.024293, -.015364, .015364, .024293, .034356] m^3/s  area_const_PB=1e-4 m^2  p_diff_TLU_const_PB=[-.1, .3, .5, .7] MPa  vol_flow_TLU_const_PB=[-.0009, .0016, .002, .0024] m^3/s  S_max_AB=7.5e-3 m  del_S_max_AB=0.005 m  area_max_AB=1e-4 m^2  del_S_TLU_AB=[0, .00125, .0025, .00375, .005] m  valve_area_TLU_AB=[1e-10, 1e-05, 4e-05, 6e-05, .0001] m^2  del_S_vol_flow_TLU_AB=[0, .00125, .0025, .00375, .005] m  p_diff_TLU_AB=[-.1, .3, .5, .7] MPa  vol_flow_TLU_AB=[-1e-08, 2.2e-08, 2.8e-08, 3.4e-08; -9e-06, .00015, .0002, .00024; -.00036, .00063, .00081, .00096; -.00054, .00094, .0012, .0014; -.00091, .0016, .002, .0024] m^3/s  area_const_AB=1e-4 m^2  p_diff_TLU_const_AB=[-.1, .3, .5, .7] MPa  vol_flow_TLU_const_AB=[-.0009, .0016, .002, .0024] m^3/s  S_max_AT=(0) - 0.0254*(valves.control.l.max) m  del_S_max_AT=(valves.control.l.max) - (valves.control.l.max)/(lines.sky.main.s.t)*(1e-9) in  area_max_AT=lines.sky.main.s.t in^2  del_S_TLU_AT=[0, .00125, .0025, .00375, .005] m  valve_area_TLU_AT=[1e-09, 2.0352e-07, 4.0736e-05, .00011438, .00034356] m^2  del_S_vol_flow_TLU_AT=[0, .00125, .0025, .00375, .005] m  p_diff_TLU_AT=[-10000000, -5000000, -2000000, 2000000, 5000000, 10000000] Pa  vol_flow_TLU_AT=[-1e-07, -7.0711e-08, -4.4721e-08, 4.4721e-08, 7.0711e-08, 1e-07; -2.0352e-05, -1.4391e-05, -9.1017e-06, 9.1017e-06, 1.4391e-05, 2.0352e-05; -.0040736, -.0028805, -.0018218, .0018218, .0028805, .0040736; -.011438, -.0080879, -.0051152, .0051152, .0080879, .011438; -.034356, -.024293, -.015364, .015364, .024293, .034356] m^3/s  area_const_AT=1e-4 m^2  p_diff_TLU_const_AT=[-.1, .3, .5, .7] MPa  vol_flow_TLU_const_AT=[-.0009, .0016, .002, .0024] m^3/s  S_max_BT=-(0) + 0.0254*(valves.control.l.max) m  del_S_max_BT=(valves.control.l.max) - (valves.control.l.max)/(lines.sky.main.s.t)*(1e-9) in  area_max_BT=lines.sky.main.s.t in^2  del_S_TLU_BT=[0, .00125, .0025, .00375, .005] m  valve_area_TLU_BT=[1e-09, 2.0352e-07, 4.0736e-05, .00011438, .00034356] m^2  del_S_vol_flow_TLU_BT=[0, .00125, .0025, .00375, .005] m  p_diff_TLU_BT=[-10000000, -5000000, -2000000, 2000000, 5000000, 10000000] Pa  vol_flow_TLU_BT=[-1e-07, -7.0711e-08, -4.4721e-08, 4.4721e-08, 7.0711e-08, 1e-07; -2.0352e-05, -1.4391e-05, -9.1017e-06, 9.1017e-06, 1.4391e-05, 2.0352e-05; -.0040736, -.0028805, -.0018218, .0018218, .0028805, .0040736; -.011438, -.0080879, -.0051152, .0051152, .0080879, .011438; -.034356, -.024293, -.015364, .015364, .024293, .034356] m^3/s  area_const_BT=1e-4 m^2  p_diff_TLU_const_BT=[-.1, .3, .5, .7] MPa  vol_flow_TLU_const_BT=[-.0009, .0016, .002, .0024] m^3/s  S_max_PT=0 m  del_S_max_PT=0.005 m  area_max_PT=1e-4 m^2  del_S_TLU_PT=[0, .00125, .0025, .00375, .005] m  valve_area_TLU_PT=[1e-10, 1e-05, 4e-05, 6e-05, .0001] m^2  del_S_vol_flow_TLU_PT=[0, .00125, .0025, .00375, .005] m  p_diff_TLU_PT=[-.1, .3, .5, .7] MPa  vol_flow_TLU_PT=[-1e-08, 2.2e-08, 2.8e-08, 3.4e-08; -9e-06, .00015, .0002, .00024; -.00036, .00063, .00081, .00096; -.00054, .00094, .0012, .0014; -.00091, .0016, .002, .0024] m^3/s
  Valve Actuator : SimscapeFluids_lib/Valve Actuators/Proportional Valve Actuator  gain=1 in  time_constant=valves.control.tau.b s  valve_stroke=valves.control.l.max in
  A : PMIOPort  Side=Right
  T : PMIOPort  Port=2  Side=Right
  s : PMIOPort  Port=3  Side=Left
  Act : PMIOPort  Port=4  Side=Left
  m : Outport
  wires:
  Bus Creator/1 -> m/1  "Lift"
  Sensor A/1 -> Bus Creator/2  "B"
  Sensor B/1 -> Bus Creator/1  "A"
  connections:
  Hose A/RConn1 -- Counterbalance Valve B/RConn1 -- Counterbalance Valve A/RConn2 -- CVHC CbValveBP/LConn1
  s/RConn1 -- Valve Actuator/LConn1
  Sensor B/LConn2 -- Counterbalance Valve A/LConn1
  Hose B/RConn1 -- Counterbalance Valve A/RConn1 -- Counterbalance Valve B/RConn2 -- CVHC CbValveBB/LConn1
  Counterbalance Valve B/LConn1 -- Sensor A/LConn2
  Cylinder/RConn2 -- Act/RConn1
  Mechanical Translational Reference/LConn1 -- Cylinder/LConn1
  Sensor B/LConn1 -- Cylinder/LConn2
  Cylinder/RConn3 -- Sensor A/LConn1
  Hose B/LConn1 -- Valve/LConn3
  Hose A/LConn1 -- Valve/LConn2
  Valve/RConn2 -- T/RConn1
  A/RConn1 -- Valve/RConn1
  Valve Actuator/RConn1 -- Valve/LConn1

== system sm_boom_lift_crawler_lib_actuators/Actuators/Sky Manifold/Sky Valves I/Boom Tilt/Lower Limit ==
  Min Spool Displacement : fl_lib/Physical Signals/Sources/PS Constant  constant=1.1e-9 m
  PS Add : fl_lib/Physical Signals/Functions/PS Add
  SLim : PMIOPort  Side=Left
  S : PMIOPort  Port=2  Side=Right
  connections:
  Min Spool Displacement/RConn1 -- PS Add/LConn2
  S/RConn1 -- PS Add/LConn1
  SLim/RConn1 -- PS Add/RConn1

== system sm_boom_lift_crawler_lib_actuators/Actuators/Sky Manifold/Sky Valves I/Tower Lift/Lower Limit ==
  Min Spool Displacement : fl_lib/Physical Signals/Sources/PS Constant  constant=1.1e-9 m
  PS Add : fl_lib/Physical Signals/Functions/PS Add
  SLim : PMIOPort  Side=Left
  S : PMIOPort  Port=2  Side=Right
  connections:
  Min Spool Displacement/RConn1 -- PS Add/LConn2
  PS Add/RConn1 -- SLim/RConn1
  S/RConn1 -- PS Add/LConn1

== system sm_boom_lift_crawler_lib_actuators/Actuators/Sky Manifold/Sky Valves II/Basket Rotate/Lower Limit ==
  Min Spool Displacement : fl_lib/Physical Signals/Sources/PS Constant  constant=1e-9 m
  PS Add : fl_lib/Physical Signals/Functions/PS Add
  S : PMIOPort  Side=Right
  SLim : PMIOPort  Port=2  Side=Left
  connections:
  S/RConn1 -- PS Add/LConn1
  PS Add/RConn1 -- SLim/RConn1
  Min Spool Displacement/RConn1 -- PS Add/LConn2
